simulink model "parcial2"  (R2020a)
settings: Solver=VariableStepAuto  StartTime=0.0  StopTime=10.0  RelTol=1e-3
settings Model: Creator=Miguel Gutierrez  LastModifiedBy=Miguel Gutierrez

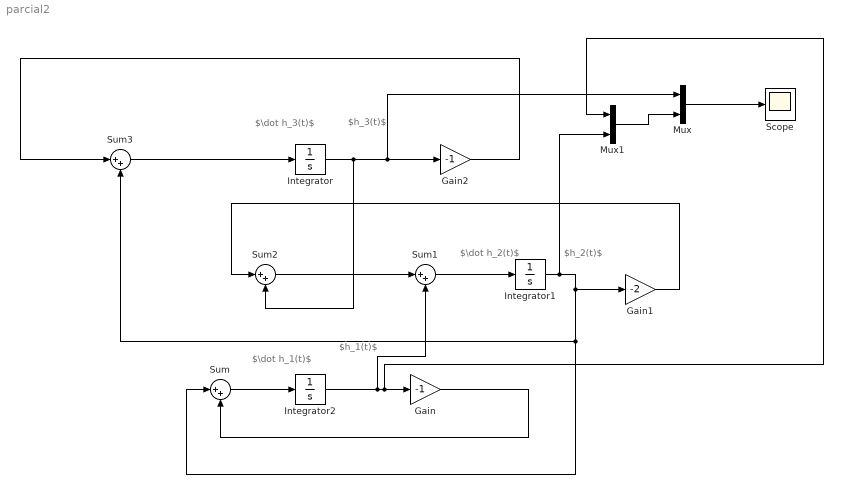
== system parcial2 ==
  note: $\dot h_3(t)$
  note: $h_3(t)$
  note: $\dot h_2(t)$
  note: $h_2(t)$
  note: $\dot h_1(t)$
  note: $h_1(t)$
  Gain : Gain  Gain=-1
  Gain1 : Gain  Gain=-2
  Gain2 : Gain  Gain=-1
  Integrator : Integrator  InitialCondition=6
  Integrator1 : Integrator  InitialCondition=7
  Integrator2 : Integrator  InitialCondition=8
  Mux : Mux  Inputs=2
  Mux1 : Mux  Inputs=2
  Scope : Scope
  Sum{,1..3} (4 alike) : Sum  Inputs=|++
  wires:
  Sum3/1 -> Integrator/1
  Integrator/1 -> Mux/1, Gain2/1, Sum2/2
  Integrator1/1 -> Mux1/2, Gain1/1, Sum3/2, Sum/1
  Sum/1 -> Integrator2/1
  Gain/1 -> Sum/2
  Gain1/1 -> Sum2/1
  Sum2/1 -> Sum1/1
  Sum1/1 -> Integrator1/1
  Gain2/1 -> Sum3/1
  Mux/1 -> Scope/1
  Mux1/1 -> Mux/2
  Integrator2/1 -> Mux1/1, Gain/1, Sum1/2
